simulink model "t06_manual_control_sol"  (R2024b)
settings: Solver=ode23t  StartTime=0.0  StopTime=inf  RelTol=1e-3  AbsTol=1e-3  EnableMultiTasking=on
model workspace (MAT data in the model file):
  A = 0.4
  Critical_Velocity = 0.01
  Damping_Factor = 1000
  Dynamic_Friction = 0.5
  Heigth_brick : Simulink.Parameter (value not decoded)
  Heigth_ramp : Simulink.Parameter (value not decoded)
  Length_brick : Simulink.Parameter (value not decoded)
  Length_ramp : Simulink.Parameter (value not decoded)
  Length_torso : Simulink.Parameter (value not decoded)
  Lower_limbs : Simulink.Parameter (value not decoded)
  Static_Friction = 0.7
  Stiffnesscoefficient = 10000
  Transition_Region_Width = 0.02
  Upper_limbs : Simulink.Parameter (value not decoded)
  Width_brick : Simulink.Parameter (value not decoded)
  Width_ramp : Simulink.Parameter (value not decoded)
  Width_torso : Simulink.Parameter (value not decoded)
  f = 1.5
  max_Joint_change = 100
  r_foot : Simulink.Parameter (value not decoded)
  sampleTime : Simulink.Parameter (value not decoded)
  t_leg : Simulink.Parameter (value not decoded)
  theta : Simulink.Parameter (value not decoded)
  transferFunVal : Simulink.Parameter (value not decoded)
symbols that are objects in the model workspace (value not decoded): Length_torso, Lower_limbs, t_leg, Upper_limbs, Width_torso
undefined symbols (not defined in the file): X, Y, Z
libraries: sm_lib x78, nesl_utility x13, functionAngles x6, functionBezier_backward x3, vrlib x1
(part 4 of 5)

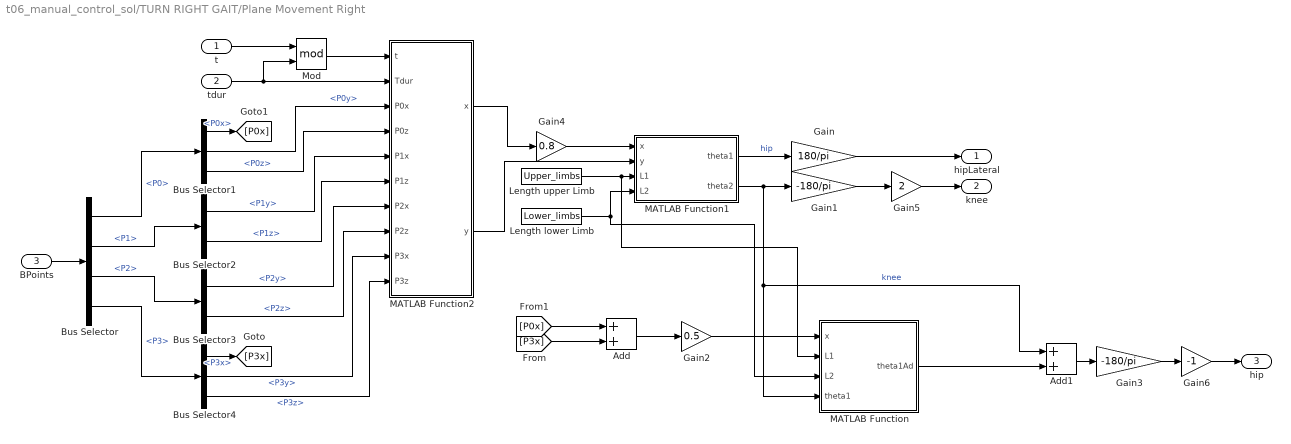
== system t06_manual_control_sol/TURN RIGHT GAIT/Plane Movement Right ==
  t : Inport
  tdur : Inport  Port=2
  BPoints : Inport  Port=3
  Add : Sum
  Add1 : Sum
  Bus Selector : BusSelector  OutputSignals=P0,P1,P2,P3
  Bus Selector1 : BusSelector  OutputSignals=P0x,P0y,P0z
  Bus Selector2 : BusSelector  OutputSignals=P1y,P1z
  Bus Selector3 : BusSelector  OutputSignals=P2y,P2z
  Bus Selector4 : BusSelector  OutputSignals=P3x,P3y,P3z
  Gain : Gain  Gain=180/pi
  Gain1 : Gain  Gain=-180/pi
  Gain2 : Gain  Gain=0.5
  Gain3 : Gain  Gain=-180/pi
  Gain4 : Gain  Gain=0.8
  Gain5 : Gain  Gain=2
  Gain6 : Gain  Gain=-1
  Length lower Limb : Constant  Value=Lower_limbs
  Length upper Limb : Constant  Value=Upper_limbs
  MATLAB Function : MATLAB Function  TreatAsAtomicUnit=on
  MATLAB Function1 : MATLAB Function  TreatAsAtomicUnit=on
  MATLAB Function2 : MATLAB Function  TreatAsAtomicUnit=on
  Mod : Math  Operator=mod
  hipLateral : Outport
  knee : Outport  Port=2
  hip : Outport  Port=3
  wires:
  Gain4/1 -> MATLAB Function1/1(x)
  Gain3/1 -> Gain6/1
  Add1/1 -> Gain3/1
  Bus Selector1/1 -> [P0x]  "<P0x>"
  Bus Selector4/1 -> [P3x]  "<P3x>"
  MATLAB Function/1(theta1Ad) -> Add1/2
  [P3x] -> Add/2
  [P0x] -> Add/1
  Add/1 -> Gain2/1
  Gain2/1 -> MATLAB Function/1(x)
  Gain/1 -> hipLateral/1
  Gain1/1 -> Gain5/1
  Length lower Limb/1 -> MATLAB Function1/4(L2), MATLAB Function/3(L2)
  Length upper Limb/1 -> MATLAB Function1/3(L1), MATLAB Function/2(L1)
  t/1 -> Mod/1
  MATLAB Function1/1(theta1) -> Gain/1  "hip"
  tdur/1 -> MATLAB Function2/2(Tdur), Mod/2
  MATLAB Function1/2(theta2) -> Gain1/1, MATLAB Function/4(theta1), Add1/1  "knee"
  MATLAB Function2/1(x) -> Gain4/1
  MATLAB Function2/2(y) -> MATLAB Function1/2(y)
  Bus Selector/3 -> Bus Selector3/1  "<P2>"
  Bus Selector3/2 -> MATLAB Function2/8(P2z)  "<P2z>"
  Bus Selector2/1 -> MATLAB Function2/5(P1x)  "<P1y>"
  Bus Selector3/1 -> MATLAB Function2/7(P2x)  "<P2y>"
  Bus Selector4/2 -> MATLAB Function2/9(P3x)  "<P3y>"
  Bus Selector1/3 -> MATLAB Function2/4(P0z)  "<P0z>"
  Bus Selector/4 -> Bus Selector4/1  "<P3>"
  Bus Selector4/3 -> MATLAB Function2/10(P3z)  "<P3z>"
  Bus Selector/2 -> Bus Selector2/1  "<P1>"
  BPoints/1 -> Bus Selector/1
  Bus Selector1/2 -> MATLAB Function2/3(P0x)  "<P0y>"
  Bus Selector/1 -> Bus Selector1/1  "<P0>"
  Bus Selector2/2 -> MATLAB Function2/6(P1z)  "<P1z>"
  Mod/1 -> MATLAB Function2/1(t)
  Gain5/1 -> knee/1
  Gain6/1 -> hip/1

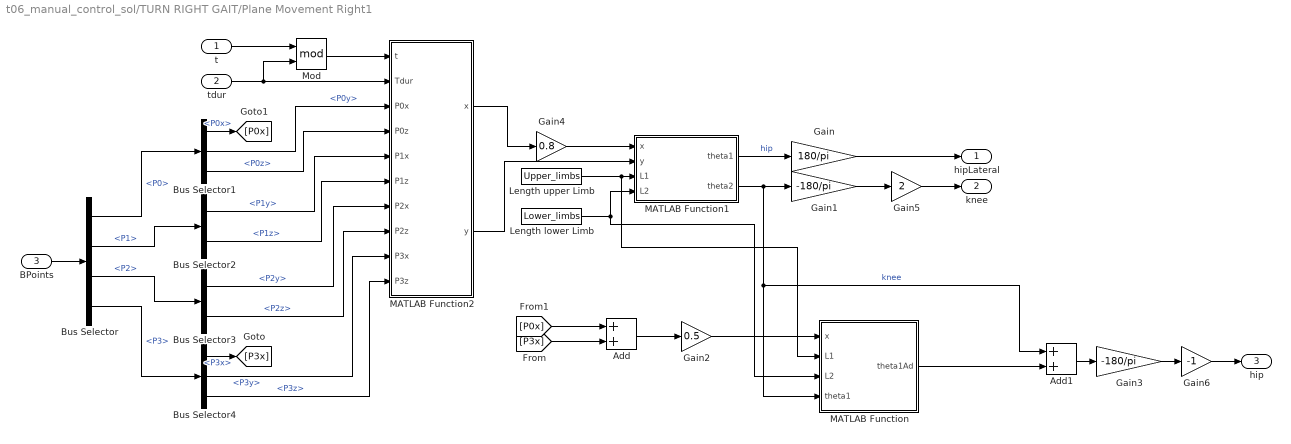
== system t06_manual_control_sol/TURN RIGHT GAIT/Plane Movement Right1 ==
  t : Inport
  tdur : Inport  Port=2
  BPoints : Inport  Port=3
  Add : Sum
  Add1 : Sum
  Bus Selector : BusSelector  OutputSignals=P0,P1,P2,P3
  Bus Selector1 : BusSelector  OutputSignals=P0x,P0y,P0z
  Bus Selector2 : BusSelector  OutputSignals=P1y,P1z
  Bus Selector3 : BusSelector  OutputSignals=P2y,P2z
  Bus Selector4 : BusSelector  OutputSignals=P3x,P3y,P3z
  Gain : Gain  Gain=180/pi
  Gain1 : Gain  Gain=-180/pi
  Gain2 : Gain  Gain=0.5
  Gain3 : Gain  Gain=-180/pi
  Gain4 : Gain  Gain=0.8
  Gain5 : Gain  Gain=2
  Gain6 : Gain  Gain=-1
  Length lower Limb : Constant  Value=Lower_limbs
  Length upper Limb : Constant  Value=Upper_limbs
  MATLAB Function : MATLAB Function  TreatAsAtomicUnit=on
  MATLAB Function1 : MATLAB Function  TreatAsAtomicUnit=on
  MATLAB Function2 : MATLAB Function  TreatAsAtomicUnit=on
  Mod : Math  Operator=mod
  hipLateral : Outport
  knee : Outport  Port=2
  hip : Outport  Port=3
  wires:
  Gain6/1 -> hip/1
  Gain5/1 -> knee/1
  Mod/1 -> MATLAB Function2/1(t)
  Bus Selector2/2 -> MATLAB Function2/6(P1z)  "<P1z>"
  Bus Selector/1 -> Bus Selector1/1  "<P0>"
  Bus Selector1/2 -> MATLAB Function2/3(P0x)  "<P0y>"
  BPoints/1 -> Bus Selector/1
  Bus Selector/2 -> Bus Selector2/1  "<P1>"
  Bus Selector4/3 -> MATLAB Function2/10(P3z)  "<P3z>"
  Bus Selector/4 -> Bus Selector4/1  "<P3>"
  Bus Selector1/3 -> MATLAB Function2/4(P0z)  "<P0z>"
  Bus Selector4/2 -> MATLAB Function2/9(P3x)  "<P3y>"
  Bus Selector3/1 -> MATLAB Function2/7(P2x)  "<P2y>"
  Bus Selector2/1 -> MATLAB Function2/5(P1x)  "<P1y>"
  Bus Selector3/2 -> MATLAB Function2/8(P2z)  "<P2z>"
  Bus Selector/3 -> Bus Selector3/1  "<P2>"
  MATLAB Function2/2(y) -> MATLAB Function1/2(y)
  MATLAB Function2/1(x) -> Gain4/1
  MATLAB Function1/2(theta2) -> Add1/1, MATLAB Function/4(theta1), Gain1/1  "knee"
  tdur/1 -> Mod/2, MATLAB Function2/2(Tdur)
  MATLAB Function1/1(theta1) -> Gain/1  "hip"
  t/1 -> Mod/1
  Length upper Limb/1 -> MATLAB Function/2(L1), MATLAB Function1/3(L1)
  Length lower Limb/1 -> MATLAB Function/3(L2), MATLAB Function1/4(L2)
  Gain1/1 -> Gain5/1
  Gain/1 -> hipLateral/1
  Gain2/1 -> MATLAB Function/1(x)
  Add/1 -> Gain2/1
  [P0x] -> Add/1
  [P3x] -> Add/2
  MATLAB Function/1(theta1Ad) -> Add1/2
  Bus Selector4/1 -> [P3x]  "<P3x>"
  Bus Selector1/1 -> [P0x]  "<P0x>"
  Add1/1 -> Gain3/1
  Gain3/1 -> Gain6/1
  Gain4/1 -> MATLAB Function1/1(x)

== system t06_manual_control_sol/TURN RIGHT GAIT/Subsystem ==
  t : Inport
  tdur : Inport  Port=2
  Add : Sum  Inputs=+-
  Add1 : Sum  Inputs=+-
  Add2 : Sum  Inputs=+-
  Gain : Gain  Gain=0.25
  Gain1 : Gain  Gain=0.5
  Gain2 : Gain  Gain=0.75
  t_0.25 : Outport
  t_0.5 : Outport  Port=2
  t_0.75 : Outport  Port=3
  wires:
  tdur/1 -> Gain/1, Gain2/1, Gain1/1
  Gain2/1 -> Add2/2
  Gain1/1 -> Add1/2
  t/1 -> Add/1, Add1/1, Add2/1
  Gain/1 -> Add/2
  Add/1 -> t_0.25/1
  Add1/1 -> t_0.5/1
  Add2/1 -> t_0.75/1

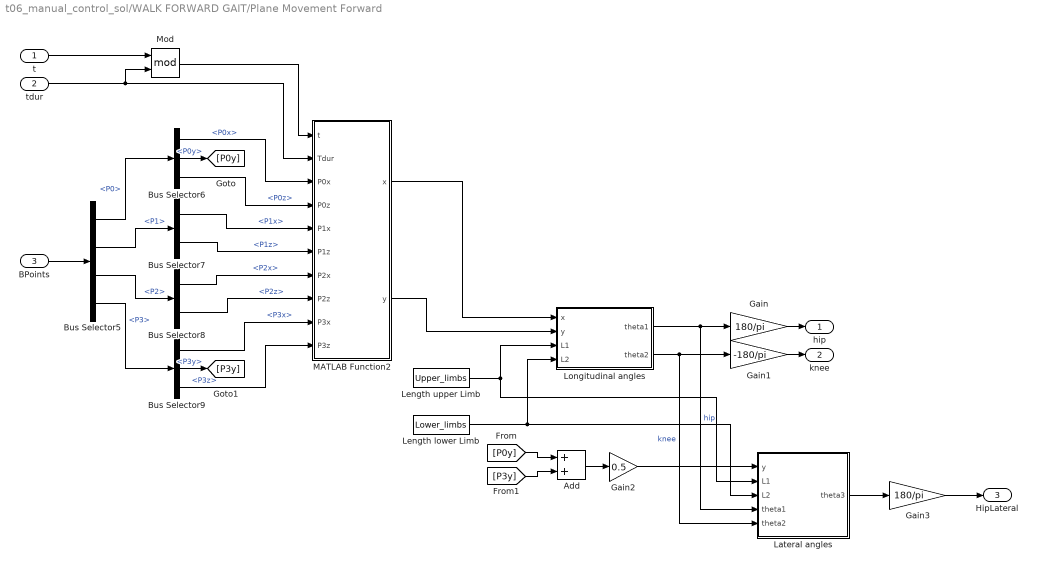
== system t06_manual_control_sol/WALK FORWARD GAIT/Plane Movement Forward ==
  t : Inport
  tdur : Inport  Port=2
  BPoints : Inport  Port=3
  Add : Sum
  Bus Selector5 : BusSelector  OutputSignals=P0,P1,P2,P3
  Bus Selector6 : BusSelector  OutputSignals=P0x,P0y,P0z
  Bus Selector7 : BusSelector  OutputSignals=P1x,P1z
  Bus Selector8 : BusSelector  OutputSignals=P2x,P2z
  Bus Selector9 : BusSelector  OutputSignals=P3x,P3y,P3z
  Gain : Gain  Gain=180/pi
  Gain1 : Gain  Gain=-180/pi
  Gain2 : Gain  Gain=0.5
  Gain3 : Gain  Gain=180/pi
  Lateral angles : MATLAB Function  TreatAsAtomicUnit=on
  Length lower Limb : Constant  Value=Lower_limbs
  Length upper Limb : Constant  Value=Upper_limbs
  Longitudinal angles : MATLAB Function  TreatAsAtomicUnit=on
  MATLAB Function2 : MATLAB Function  TreatAsAtomicUnit=on
  Mod : Math  Operator=mod
  hip : Outport
  knee : Outport  Port=2
  HipLateral : Outport  Port=3
  wires:
  Gain3/1 -> HipLateral/1
  Lateral angles/1(theta3) -> Gain3/1
  [P3y] -> Add/2
  [P0y] -> Add/1
  Bus Selector9/2 -> [P3y]  "<P3y>"
  Bus Selector6/2 -> [P0y]  "<P0y>"
  Gain2/1 -> Lateral angles/1(y)
  Add/1 -> Gain2/1
  Gain/1 -> hip/1
  Gain1/1 -> knee/1
  Length lower Limb/1 -> Lateral angles/3(L2), Longitudinal angles/4(L2)
  Length upper Limb/1 -> Lateral angles/2(L1), Longitudinal angles/3(L1)
  t/1 -> Mod/1
  Longitudinal angles/1(theta1) -> Gain/1, Lateral angles/4(theta1)  "hip"
  tdur/1 -> Mod/2, MATLAB Function2/2(Tdur)
  Longitudinal angles/2(theta2) -> Lateral angles/5(theta2), Gain1/1  "knee"
  MATLAB Function2/1(x) -> Longitudinal angles/1(x)
  MATLAB Function2/2(y) -> Longitudinal angles/2(y)
  Bus Selector5/3 -> Bus Selector8/1  "<P2>"
  Bus Selector8/2 -> MATLAB Function2/8(P2z)  "<P2z>"
  Bus Selector7/1 -> MATLAB Function2/5(P1x)  "<P1x>"
  Bus Selector8/1 -> MATLAB Function2/7(P2x)  "<P2x>"
  Bus Selector9/1 -> MATLAB Function2/9(P3x)  "<P3x>"
  Bus Selector6/3 -> MATLAB Function2/4(P0z)  "<P0z>"
  Bus Selector5/4 -> Bus Selector9/1  "<P3>"
  Bus Selector9/3 -> MATLAB Function2/10(P3z)  "<P3z>"
  Bus Selector5/2 -> Bus Selector7/1  "<P1>"
  BPoints/1 -> Bus Selector5/1
  Bus Selector6/1 -> MATLAB Function2/3(P0x)  "<P0x>"
  Bus Selector5/1 -> Bus Selector6/1  "<P0>"
  Bus Selector7/2 -> MATLAB Function2/6(P1z)  "<P1z>"
  Mod/1 -> MATLAB Function2/1(t)

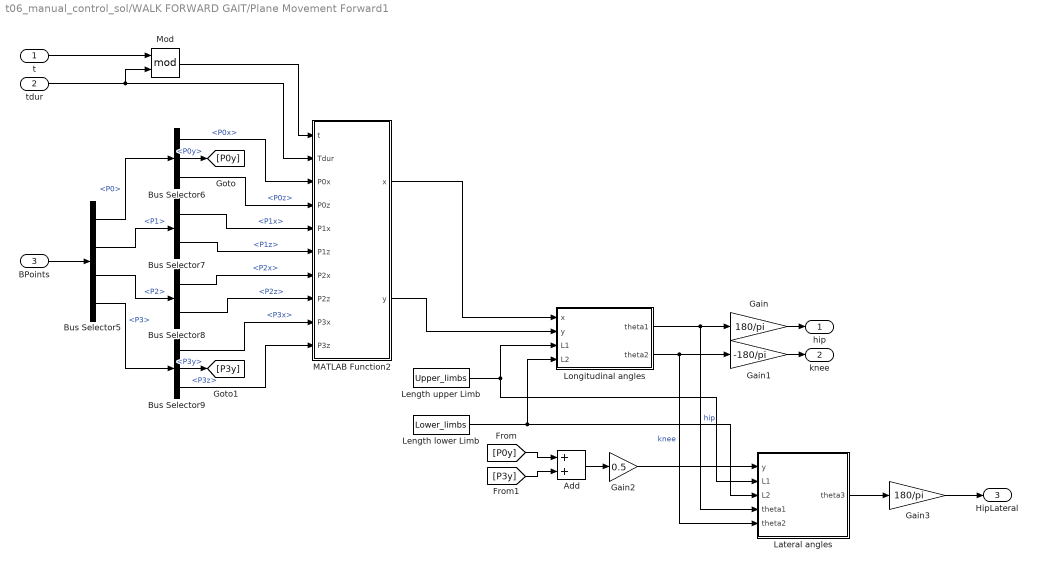
== system t06_manual_control_sol/WALK FORWARD GAIT/Plane Movement Forward1 ==
  t : Inport
  tdur : Inport  Port=2
  BPoints : Inport  Port=3
  Add : Sum
  Bus Selector5 : BusSelector  OutputSignals=P0,P1,P2,P3
  Bus Selector6 : BusSelector  OutputSignals=P0x,P0y,P0z
  Bus Selector7 : BusSelector  OutputSignals=P1x,P1z
  Bus Selector8 : BusSelector  OutputSignals=P2x,P2z
  Bus Selector9 : BusSelector  OutputSignals=P3x,P3y,P3z
  Gain : Gain  Gain=180/pi
  Gain1 : Gain  Gain=-180/pi
  Gain2 : Gain  Gain=0.5
  Gain3 : Gain  Gain=180/pi
  Lateral angles : MATLAB Function  TreatAsAtomicUnit=on
  Length lower Limb : Constant  Value=Lower_limbs
  Length upper Limb : Constant  Value=Upper_limbs
  Longitudinal angles : MATLAB Function  TreatAsAtomicUnit=on
  MATLAB Function2 : MATLAB Function  TreatAsAtomicUnit=on
  Mod : Math  Operator=mod
  hip : Outport
  knee : Outport  Port=2
  HipLateral : Outport  Port=3
  wires:
  Gain3/1 -> HipLateral/1
  Lateral angles/1(theta3) -> Gain3/1
  [P3y] -> Add/2
  [P0y] -> Add/1
  Bus Selector9/2 -> [P3y]  "<P3y>"
  Bus Selector6/2 -> [P0y]  "<P0y>"
  Gain2/1 -> Lateral angles/1(y)
  Add/1 -> Gain2/1
  Gain/1 -> hip/1
  Gain1/1 -> knee/1
  Length lower Limb/1 -> Lateral angles/3(L2), Longitudinal angles/4(L2)
  Length upper Limb/1 -> Lateral angles/2(L1), Longitudinal angles/3(L1)
  t/1 -> Mod/1
  Longitudinal angles/1(theta1) -> Gain/1, Lateral angles/4(theta1)  "hip"
  tdur/1 -> Mod/2, MATLAB Function2/2(Tdur)
  Longitudinal angles/2(theta2) -> Lateral angles/5(theta2), Gain1/1  "knee"
  MATLAB Function2/1(x) -> Longitudinal angles/1(x)
  MATLAB Function2/2(y) -> Longitudinal angles/2(y)
  Bus Selector5/3 -> Bus Selector8/1  "<P2>"
  Bus Selector8/2 -> MATLAB Function2/8(P2z)  "<P2z>"
  Bus Selector7/1 -> MATLAB Function2/5(P1x)  "<P1x>"
  Bus Selector8/1 -> MATLAB Function2/7(P2x)  "<P2x>"
  Bus Selector9/1 -> MATLAB Function2/9(P3x)  "<P3x>"
  Bus Selector6/3 -> MATLAB Function2/4(P0z)  "<P0z>"
  Bus Selector5/4 -> Bus Selector9/1  "<P3>"
  Bus Selector9/3 -> MATLAB Function2/10(P3z)  "<P3z>"
  Bus Selector5/2 -> Bus Selector7/1  "<P1>"
  BPoints/1 -> Bus Selector5/1
  Bus Selector6/1 -> MATLAB Function2/3(P0x)  "<P0x>"
  Bus Selector5/1 -> Bus Selector6/1  "<P0>"
  Bus Selector7/2 -> MATLAB Function2/6(P1z)  "<P1z>"
  Mod/1 -> MATLAB Function2/1(t)

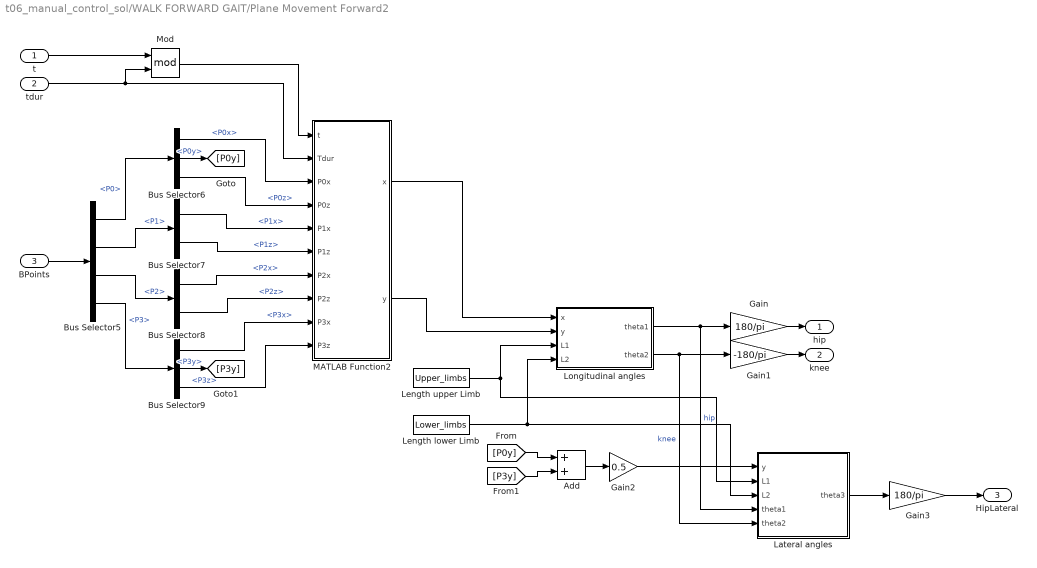
== system t06_manual_control_sol/WALK FORWARD GAIT/Plane Movement Forward2 ==
  t : Inport
  tdur : Inport  Port=2
  BPoints : Inport  Port=3
  Add : Sum
  Bus Selector5 : BusSelector  OutputSignals=P0,P1,P2,P3
  Bus Selector6 : BusSelector  OutputSignals=P0x,P0y,P0z
  Bus Selector7 : BusSelector  OutputSignals=P1x,P1z
  Bus Selector8 : BusSelector  OutputSignals=P2x,P2z
  Bus Selector9 : BusSelector  OutputSignals=P3x,P3y,P3z
  Gain : Gain  Gain=180/pi
  Gain1 : Gain  Gain=-180/pi
  Gain2 : Gain  Gain=0.5
  Gain3 : Gain  Gain=180/pi
  Lateral angles : MATLAB Function  TreatAsAtomicUnit=on
  Length lower Limb : Constant  Value=Lower_limbs
  Length upper Limb : Constant  Value=Upper_limbs
  Longitudinal angles : MATLAB Function  TreatAsAtomicUnit=on
  MATLAB Function2 : MATLAB Function  TreatAsAtomicUnit=on
  Mod : Math  Operator=mod
  hip : Outport
  knee : Outport  Port=2
  HipLateral : Outport  Port=3
  wires:
  Gain3/1 -> HipLateral/1
  Lateral angles/1(theta3) -> Gain3/1
  [P3y] -> Add/2
  [P0y] -> Add/1
  Bus Selector9/2 -> [P3y]  "<P3y>"
  Bus Selector6/2 -> [P0y]  "<P0y>"
  Gain2/1 -> Lateral angles/1(y)
  Add/1 -> Gain2/1
  Gain/1 -> hip/1
  Gain1/1 -> knee/1
  Length lower Limb/1 -> Lateral angles/3(L2), Longitudinal angles/4(L2)
  Length upper Limb/1 -> Lateral angles/2(L1), Longitudinal angles/3(L1)
  t/1 -> Mod/1
  Longitudinal angles/1(theta1) -> Gain/1, Lateral angles/4(theta1)  "hip"
  tdur/1 -> Mod/2, MATLAB Function2/2(Tdur)
  Longitudinal angles/2(theta2) -> Lateral angles/5(theta2), Gain1/1  "knee"
  MATLAB Function2/1(x) -> Longitudinal angles/1(x)
  MATLAB Function2/2(y) -> Longitudinal angles/2(y)
  Bus Selector5/3 -> Bus Selector8/1  "<P2>"
  Bus Selector8/2 -> MATLAB Function2/8(P2z)  "<P2z>"
  Bus Selector7/1 -> MATLAB Function2/5(P1x)  "<P1x>"
  Bus Selector8/1 -> MATLAB Function2/7(P2x)  "<P2x>"
  Bus Selector9/1 -> MATLAB Function2/9(P3x)  "<P3x>"
  Bus Selector6/3 -> MATLAB Function2/4(P0z)  "<P0z>"
  Bus Selector5/4 -> Bus Selector9/1  "<P3>"
  Bus Selector9/3 -> MATLAB Function2/10(P3z)  "<P3z>"
  Bus Selector5/2 -> Bus Selector7/1  "<P1>"
  BPoints/1 -> Bus Selector5/1
  Bus Selector6/1 -> MATLAB Function2/3(P0x)  "<P0x>"
  Bus Selector5/1 -> Bus Selector6/1  "<P0>"
  Bus Selector7/2 -> MATLAB Function2/6(P1z)  "<P1z>"
  Mod/1 -> MATLAB Function2/1(t)

== system t06_manual_control_sol/WALK FORWARD GAIT/Plane Movement Forward3 ==
  t : Inport
  tdur : Inport  Port=2
  BPoints : Inport  Port=3
  Add : Sum
  Bus Selector5 : BusSelector  OutputSignals=P0,P1,P2,P3
  Bus Selector6 : BusSelector  OutputSignals=P0x,P0y,P0z
  Bus Selector7 : BusSelector  OutputSignals=P1x,P1z
  Bus Selector8 : BusSelector  OutputSignals=P2x,P2z
  Bus Selector9 : BusSelector  OutputSignals=P3x,P3y,P3z
  Gain : Gain  Gain=180/pi
  Gain1 : Gain  Gain=-180/pi
  Gain2 : Gain  Gain=0.5
  Gain3 : Gain  Gain=180/pi
  Lateral angles : MATLAB Function  TreatAsAtomicUnit=on
  Length lower Limb : Constant  Value=Lower_limbs
  Length upper Limb : Constant  Value=Upper_limbs
  Longitudinal angles : MATLAB Function  TreatAsAtomicUnit=on
  MATLAB Function2 : MATLAB Function  TreatAsAtomicUnit=on
  Mod : Math  Operator=mod
  hip : Outport
  knee : Outport  Port=2
  HipLateral : Outport  Port=3
  wires:
  Gain3/1 -> HipLateral/1
  Lateral angles/1(theta3) -> Gain3/1
  [P3y] -> Add/2
  [P0y] -> Add/1
  Bus Selector9/2 -> [P3y]  "<P3y>"
  Bus Selector6/2 -> [P0y]  "<P0y>"
  Gain2/1 -> Lateral angles/1(y)
  Add/1 -> Gain2/1
  Gain/1 -> hip/1
  Gain1/1 -> knee/1
  Length lower Limb/1 -> Lateral angles/3(L2), Longitudinal angles/4(L2)
  Length upper Limb/1 -> Lateral angles/2(L1), Longitudinal angles/3(L1)
  t/1 -> Mod/1
  Longitudinal angles/1(theta1) -> Gain/1, Lateral angles/4(theta1)  "hip"
  tdur/1 -> Mod/2, MATLAB Function2/2(Tdur)
  Longitudinal angles/2(theta2) -> Lateral angles/5(theta2), Gain1/1  "knee"
  MATLAB Function2/1(x) -> Longitudinal angles/1(x)
  MATLAB Function2/2(y) -> Longitudinal angles/2(y)
  Bus Selector5/3 -> Bus Selector8/1  "<P2>"
  Bus Selector8/2 -> MATLAB Function2/8(P2z)  "<P2z>"
  Bus Selector7/1 -> MATLAB Function2/5(P1x)  "<P1x>"
  Bus Selector8/1 -> MATLAB Function2/7(P2x)  "<P2x>"
  Bus Selector9/1 -> MATLAB Function2/9(P3x)  "<P3x>"
  Bus Selector6/3 -> MATLAB Function2/4(P0z)  "<P0z>"
  Bus Selector5/4 -> Bus Selector9/1  "<P3>"
  Bus Selector9/3 -> MATLAB Function2/10(P3z)  "<P3z>"
  Bus Selector5/2 -> Bus Selector7/1  "<P1>"
  BPoints/1 -> Bus Selector5/1
  Bus Selector6/1 -> MATLAB Function2/3(P0x)  "<P0x>"
  Bus Selector5/1 -> Bus Selector6/1  "<P0>"
  Bus Selector7/2 -> MATLAB Function2/6(P1z)  "<P1z>"
  Mod/1 -> MATLAB Function2/1(t)

== system t06_manual_control_sol/WALK FORWARD GAIT/Subsystem ==
  t : Inport
  tdur : Inport  Port=2
  Add : Sum  Inputs=+-
  Add1 : Sum  Inputs=+-
  Add2 : Sum  Inputs=+-
  Gain : Gain  Gain=0.25
  Gain1 : Gain  Gain=0.5
  Gain2 : Gain  Gain=0.75
  t_0.25 : Outport
  t_0.5 : Outport  Port=2
  t_0.75 : Outport  Port=3
  wires:
  tdur/1 -> Gain/1, Gain2/1, Gain1/1
  Gain2/1 -> Add2/2
  Gain1/1 -> Add1/2
  t/1 -> Add/1, Add1/1, Add2/1
  Gain/1 -> Add/2
  Add/1 -> t_0.25/1
  Add1/1 -> t_0.5/1
  Add2/1 -> t_0.75/1

== system t06_manual_control_sol/Walk Back Gait - Bezier Curves/Plane Movement BL ==
  t : Inport
  tdur : Inport  Port=2
  BPoints : Inport  Port=3
  Add : Sum
  Bus Selector : BusSelector  OutputSignals=P0,P1,P2,P3
  Bus Selector1 : BusSelector  OutputSignals=P0x,P0y,P0z
  Bus Selector2 : BusSelector  OutputSignals=P1x,P1z
  Bus Selector3 : BusSelector  OutputSignals=P2x,P2z
  Bus Selector4 : BusSelector  OutputSignals=P3x,P3y,P3z
  Gain : Gain  Gain=180/pi
  Gain1 : Gain  Gain=-180/pi
  Gain2 : Gain  Gain=0.5
  Gain3 : Gain  Gain=180/pi
  Length lower Limb : Constant  Value=Lower_limbs
  Length upper Limb : Constant  Value=Upper_limbs
  MATLAB : functionAngles/MATLAB  SystemSampleTime=-1  VariantActivationTime=update diagram  AllowFlexibleInterface=on  Latency=0  AutoFrameSizeCalculation=off
  MATLAB Function : functionAngles/MATLAB Function  SystemSampleTime=-1  VariantActivationTime=update diagram  AllowFlexibleInterface=on  Latency=0  AutoFrameSizeCalculation=off
  MATLAB Function2 : functionBezier_backward/MATLAB Function2  SystemSampleTime=-1  VariantActivationTime=update diagram  AllowFlexibleInterface=on  Latency=0  AutoFrameSizeCalculation=off
  Mod : Math  Operator=mod
  hip : Outport
  knee : Outport  Port=2
  hipLateral : Outport  Port=3
  wires:
  MATLAB Function/1 -> Gain3/1
  Gain3/1 -> hipLateral/1
  Bus Selector4/2 -> [P3y]  "<P3y>"
  Bus Selector1/2 -> [P0y]  "<P0y>"
  Gain2/1 -> MATLAB Function/1
  [P3y] -> Add/2
  Add/1 -> Gain2/1
  [P0y] -> Add/1
  MATLAB Function2/2 -> MATLAB/2
  MATLAB Function2/1 -> MATLAB/1
  MATLAB/2 -> Gain1/1, MATLAB Function/5  "knee"
  tdur/1 -> Mod/2, MATLAB Function2/2
  MATLAB/1 -> Gain/1, MATLAB Function/4  "hip"
  Length upper Limb/1 -> MATLAB Function/2, MATLAB/3
  Length lower Limb/1 -> MATLAB/4, MATLAB Function/3
  Gain1/1 -> knee/1
  Gain/1 -> hip/1
  Bus Selector/3 -> Bus Selector3/1  "<P2>"
  Bus Selector3/2 -> MATLAB Function2/8  "<P2z>"
  Bus Selector2/1 -> MATLAB Function2/5  "<P1x>"
  Bus Selector3/1 -> MATLAB Function2/7  "<P2x>"
  Bus Selector4/1 -> MATLAB Function2/9  "<P3x>"
  Bus Selector1/3 -> MATLAB Function2/4  "<P0z>"
  Bus Selector/4 -> Bus Selector4/1  "<P3>"
  Bus Selector4/3 -> MATLAB Function2/10  "<P3z>"
  Bus Selector/2 -> Bus Selector2/1  "<P1>"
  BPoints/1 -> Bus Selector/1
  Bus Selector1/1 -> MATLAB Function2/3  "<P0x>"
  Bus Selector/1 -> Bus Selector1/1  "<P0>"
  Bus Selector2/2 -> MATLAB Function2/6  "<P1z>"
  t/1 -> Mod/1
  Mod/1 -> MATLAB Function2/1

== system t06_manual_control_sol/Walk Back Gait - Bezier Curves/Plane Movement BR ==
  t : Inport
  tdur : Inport  Port=2
  BPoints : Inport  Port=3
  Add : Sum
  Bus Selector : BusSelector  OutputSignals=P0,P1,P2,P3
  Bus Selector1 : BusSelector  OutputSignals=P0x,P0y,P0z
  Bus Selector2 : BusSelector  OutputSignals=P1x,P1z
  Bus Selector3 : BusSelector  OutputSignals=P2x,P2z
  Bus Selector4 : BusSelector  OutputSignals=P3x,P3y,P3z
  Gain : Gain  Gain=180/pi
  Gain1 : Gain  Gain=-180/pi
  Gain2 : Gain  Gain=0.5
  Gain3 : Gain  Gain=180/pi
  Length lower Limb : Constant  Value=Lower_limbs
  Length upper Limb : Constant  Value=Upper_limbs
  MATLAB : functionAngles/MATLAB  SystemSampleTime=-1  VariantActivationTime=update diagram  AllowFlexibleInterface=on  Latency=0  AutoFrameSizeCalculation=off
  MATLAB Function : functionAngles/MATLAB Function  SystemSampleTime=-1  VariantActivationTime=update diagram  AllowFlexibleInterface=on  Latency=0  AutoFrameSizeCalculation=off
  MATLAB Function2 : functionBezier_backward/MATLAB Function2  SystemSampleTime=-1  VariantActivationTime=update diagram  AllowFlexibleInterface=on  Latency=0  AutoFrameSizeCalculation=off
  Mod : Math  Operator=mod
  hip : Outport
  knee : Outport  Port=2
  hipLateral : Outport  Port=3
  wires:
  MATLAB Function/1 -> Gain3/1
  Gain3/1 -> hipLateral/1
  Bus Selector4/2 -> [P3y]  "<P3y>"
  Bus Selector1/2 -> [P0y]  "<P0y>"
  Gain2/1 -> MATLAB Function/1
  [P3y] -> Add/2
  Add/1 -> Gain2/1
  [P0y] -> Add/1
  MATLAB Function2/2 -> MATLAB/2
  MATLAB Function2/1 -> MATLAB/1
  MATLAB/2 -> Gain1/1, MATLAB Function/5  "knee"
  tdur/1 -> MATLAB Function2/2, Mod/2
  MATLAB/1 -> Gain/1, MATLAB Function/4  "hip"
  Length upper Limb/1 -> MATLAB Function/2, MATLAB/3
  Length lower Limb/1 -> MATLAB/4, MATLAB Function/3
  Gain1/1 -> knee/1
  Gain/1 -> hip/1
  Bus Selector/3 -> Bus Selector3/1  "<P2>"
  Bus Selector3/2 -> MATLAB Function2/8  "<P2z>"
  Bus Selector2/1 -> MATLAB Function2/5  "<P1x>"
  Bus Selector3/1 -> MATLAB Function2/7  "<P2x>"
  Bus Selector4/1 -> MATLAB Function2/9  "<P3x>"
  Bus Selector1/3 -> MATLAB Function2/4  "<P0z>"
  Bus Selector/4 -> Bus Selector4/1  "<P3>"
  Bus Selector4/3 -> MATLAB Function2/10  "<P3z>"
  Bus Selector/2 -> Bus Selector2/1  "<P1>"
  BPoints/1 -> Bus Selector/1
  Bus Selector1/1 -> MATLAB Function2/3  "<P0x>"
  Bus Selector/1 -> Bus Selector1/1  "<P0>"
  Bus Selector2/2 -> MATLAB Function2/6  "<P1z>"
  t/1 -> Mod/1
  Mod/1 -> MATLAB Function2/1

== system t06_manual_control_sol/Walk Back Gait - Bezier Curves/Plane Movement FL ==
  t : Inport
  tdur : Inport  Port=2
  BPoints : Inport  Port=3
  Add : Sum
  Bus Selector : BusSelector  OutputSignals=P0,P1,P2,P3
  Bus Selector1 : BusSelector  OutputSignals=P0x,P0y,P0z
  Bus Selector2 : BusSelector  OutputSignals=P1x,P1z
  Bus Selector3 : BusSelector  OutputSignals=P2x,P2z
  Bus Selector4 : BusSelector  OutputSignals=P3x,P3y,P3z
  Gain : Gain  Gain=180/pi
  Gain1 : Gain  Gain=-180/pi
  Gain2 : Gain  Gain=0.5
  Gain3 : Gain  Gain=180/pi
  Length lower Limb : Constant  Value=Lower_limbs
  Length upper Limb : Constant  Value=Upper_limbs
  MATLAB : MATLAB Function  TreatAsAtomicUnit=on
  MATLAB Function : MATLAB Function  TreatAsAtomicUnit=on
  MATLAB Function2 : MATLAB Function  TreatAsAtomicUnit=on
  Mod : Math  Operator=mod
  hip : Outport
  knee : Outport  Port=2
  hipLateral : Outport  Port=3
  wires:
  MATLAB Function/1(theta3) -> Gain3/1
  Gain3/1 -> hipLateral/1
  Bus Selector4/2 -> [P3y]  "<P3y>"
  Bus Selector1/2 -> [P0y]  "<P0y>"
  Gain2/1 -> MATLAB Function/1(y)
  [P3y] -> Add/2
  Add/1 -> Gain2/1
  [P0y] -> Add/1
  MATLAB Function2/2(y) -> MATLAB/2(y)
  MATLAB Function2/1(x) -> MATLAB/1(x)
  MATLAB/2(theta2) -> Gain1/1, MATLAB Function/5(theta2)  "knee"
  tdur/1 -> Mod/2, MATLAB Function2/2(Tdur)
  MATLAB/1(theta1) -> Gain/1, MATLAB Function/4(theta1)  "hip"
  Length upper Limb/1 -> MATLAB Function/2(L1), MATLAB/3(L1)
  Length lower Limb/1 -> MATLAB/4(L2), MATLAB Function/3(L2)
  Gain1/1 -> knee/1
  Gain/1 -> hip/1
  Bus Selector/3 -> Bus Selector3/1  "<P2>"
  Bus Selector3/2 -> MATLAB Function2/8(P2z)  "<P2z>"
  Bus Selector2/1 -> MATLAB Function2/5(P1x)  "<P1x>"
  Bus Selector3/1 -> MATLAB Function2/7(P2x)  "<P2x>"
  Bus Selector4/1 -> MATLAB Function2/9(P3x)  "<P3x>"
  Bus Selector1/3 -> MATLAB Function2/4(P0z)  "<P0z>"
  Bus Selector/4 -> Bus Selector4/1  "<P3>"
  Bus Selector4/3 -> MATLAB Function2/10(P3z)  "<P3z>"
  Bus Selector/2 -> Bus Selector2/1  "<P1>"
  BPoints/1 -> Bus Selector/1
  Bus Selector1/1 -> MATLAB Function2/3(P0x)  "<P0x>"
  Bus Selector/1 -> Bus Selector1/1  "<P0>"
  Bus Selector2/2 -> MATLAB Function2/6(P1z)  "<P1z>"
  Mod/1 -> MATLAB Function2/1(t)
  t/1 -> Mod/1

== system t06_manual_control_sol/Walk Back Gait - Bezier Curves/Plane Movement FR ==
  t : Inport
  tdur : Inport  Port=2
  BPoints : Inport  Port=3
  Add : Sum
  Bus Selector : BusSelector  OutputSignals=P0,P1,P2,P3
  Bus Selector1 : BusSelector  OutputSignals=P0x,P0y,P0z
  Bus Selector2 : BusSelector  OutputSignals=P1x,P1z
  Bus Selector3 : BusSelector  OutputSignals=P2x,P2z
  Bus Selector4 : BusSelector  OutputSignals=P3x,P3y,P3z
  Gain : Gain  Gain=180/pi
  Gain1 : Gain  Gain=-180/pi
  Gain2 : Gain  Gain=0.5
  Gain3 : Gain  Gain=180/pi
  Length lower Limb : Constant  Value=Lower_limbs
  Length upper Limb : Constant  Value=Upper_limbs
  MATLAB : functionAngles/MATLAB  SystemSampleTime=-1  VariantActivationTime=update diagram  AllowFlexibleInterface=on  Latency=0  AutoFrameSizeCalculation=off
  MATLAB Function : functionAngles/MATLAB Function  SystemSampleTime=-1  VariantActivationTime=update diagram  AllowFlexibleInterface=on  Latency=0  AutoFrameSizeCalculation=off
  MATLAB Function2 : functionBezier_backward/MATLAB Function2  SystemSampleTime=-1  VariantActivationTime=update diagram  AllowFlexibleInterface=on  Latency=0  AutoFrameSizeCalculation=off
  Mod : Math  Operator=mod
  hip : Outport
  knee : Outport  Port=2
  hipLateral : Outport  Port=3
  wires:
  MATLAB Function/1 -> Gain3/1
  Gain3/1 -> hipLateral/1
  Bus Selector4/2 -> [P3y]  "<P3y>"
  Bus Selector1/2 -> [P0y]  "<P0y>"
  Gain2/1 -> MATLAB Function/1
  [P3y] -> Add/2
  Add/1 -> Gain2/1
  [P0y] -> Add/1
  MATLAB Function2/2 -> MATLAB/2
  MATLAB Function2/1 -> MATLAB/1
  MATLAB/2 -> Gain1/1, MATLAB Function/5  "knee"
  tdur/1 -> Mod/2, MATLAB Function2/2
  MATLAB/1 -> Gain/1, MATLAB Function/4  "hip"
  Length upper Limb/1 -> MATLAB Function/2, MATLAB/3
  Length lower Limb/1 -> MATLAB/4, MATLAB Function/3
  Gain1/1 -> knee/1
  Gain/1 -> hip/1
  Bus Selector/3 -> Bus Selector3/1  "<P2>"
  Bus Selector3/2 -> MATLAB Function2/8  "<P2z>"
  Bus Selector2/1 -> MATLAB Function2/5  "<P1x>"
  Bus Selector3/1 -> MATLAB Function2/7  "<P2x>"
  Bus Selector4/1 -> MATLAB Function2/9  "<P3x>"
  Bus Selector1/3 -> MATLAB Function2/4  "<P0z>"
  Bus Selector/4 -> Bus Selector4/1  "<P3>"
  Bus Selector4/3 -> MATLAB Function2/10  "<P3z>"
  Bus Selector/2 -> Bus Selector2/1  "<P1>"
  BPoints/1 -> Bus Selector/1
  Bus Selector1/1 -> MATLAB Function2/3  "<P0x>"
  Bus Selector/1 -> Bus Selector1/1  "<P0>"
  Bus Selector2/2 -> MATLAB Function2/6  "<P1z>"
  t/1 -> Mod/1
  Mod/1 -> MATLAB Function2/1

== system t06_manual_control_sol/Walk Back Gait - Bezier Curves/Subsystem1 ==
  t : Inport
  tdur : Inport  Port=2
  Add : Sum  Inputs=+-
  Add1 : Sum  Inputs=+-
  Add2 : Sum  Inputs=+-
  Gain : Gain  Gain=0.25
  Gain1 : Gain  Gain=0.5
  Gain2 : Gain  Gain=0.75
  t_0.25 : Outport
  t_0.5 : Outport  Port=2
  t_0.75 : Outport  Port=3
  wires:
  tdur/1 -> Gain/1, Gain2/1, Gain1/1
  Gain2/1 -> Add2/2
  Gain1/1 -> Add1/2
  t/1 -> Add/1, Add1/1, Add2/1
  Gain/1 -> Add/2
  Add/1 -> t_0.25/1
  Add1/1 -> t_0.5/1
  Add2/1 -> t_0.75/1

== matlab function t06_manual_control_sol/TURN RIGHT GAIT/Plane Movement Left1/MATLAB Function1 ==
  data: x input; theta1 output; y input; L1 input; L2 input; theta2 output
function [theta1, theta2] = angSide(x,y,L1,L2)
theta1 = atan(-x/y);
if theta1 ~= 0
    d = x / (2*sin(theta1));
    theta2 = acos(d/L1);
else
    d = -y/2;
    theta2 = acos(d/L1);
end
end

== matlab function t06_manual_control_sol/WALK FORWARD GAIT/Plane Movement Forward1/Lateral angles ==
  data: y input; theta3 output; L1 input; L2 input; theta1 input; theta2 input
function theta3 = latAng(y, L1, L2, theta1, theta2)

l = cos(theta1)*(L1 + L2*cos(theta2));

theta3 = asin(y/l);

== matlab function t06_manual_control_sol/Stand Still/Plane Movement BL/Longitudinal angles ==
  data: x input; theta1 output; y input; L1 input; L2 input; theta2 output
function [theta1, theta2] = ang(x,y,L1,L2)
x;
y;
(x.^2+y.^2-L1.^2-L2.^2) / (2*L1*L2);
theta2 = acos((x.^2+y.^2-L1.^2-L2.^2) / (2*L1*L2));
beta = asin((L2*sin(theta2))./((x.^2+y.^2).^0.5));
theta1 = asin(x./((x.^2+y.^2).^0.5)) + beta;
end

== matlab function t06_manual_control_sol/Stand Still/Plane Movement BL/Lateral joint angle ==
  data: y input; theta3 output; L1 input; L2 input; theta1 input; theta2 input
function theta3 = latAng(y, L1, L2, theta1, theta2)

l = cos(theta1)*(L1 + L2*cos(theta2));

theta3 = asin(y/l);

== matlab function t06_manual_control_sol/Stand Still/Plane Movement BR/Longitudinal angles ==
  data: x input; theta1 output; y input; L1 input; L2 input; theta2 output
function [theta1, theta2] = ang(x,y,L1,L2)
x;
y;
(x.^2+y.^2-L1.^2-L2.^2) / (2*L1*L2);
theta2 = acos((x.^2+y.^2-L1.^2-L2.^2) / (2*L1*L2));
beta = asin((L2*sin(theta2))./((x.^2+y.^2).^0.5));
theta1 = asin(x./((x.^2+y.^2).^0.5)) + beta;
end

== matlab function t06_manual_control_sol/Stand Still/Plane Movement BR/Lateral joint angle ==
  data: y input; theta3 output; L1 input; L2 input; theta1 input; theta2 input
function theta3 = latAng(y, L1, L2, theta1, theta2)

l = cos(theta1)*(L1 + L2*cos(theta2));

theta3 = asin(y/l);

== matlab function t06_manual_control_sol/TURN RIGHT GAIT/Plane Movement Right1/MATLAB Function ==
  data: x input; theta1Ad output; L1 input; L2 input; theta1 input
function theta1Ad = angAd(x, L1, L2, theta1)

l = cos(theta1)*(L1 + L2);

theta1Ad = asin(-x/l);

== matlab function t06_manual_control_sol/Stand Still/Plane Movement FL/Lateral joint angle ==
  data: y input; theta3 output; L1 input; L2 input; theta1 input; theta2 input
function theta3 = latAng(y, L1, L2, theta1, theta2)

l = cos(theta1)*(L1 + L2*cos(theta2));

theta3 = asin(y/l);

== matlab function t06_manual_control_sol/Stand Still/Plane Movement FR/Lateral joint angle ==
  data: y input; theta3 output; L1 input; L2 input; theta1 input; theta2 input
function theta3 = latAng(y, L1, L2, theta1, theta2)

l = cos(theta1)*(L1 + L2*cos(theta2));

theta3 = asin(y/l);

== matlab function t06_manual_control_sol/Stand Still/Plane Movement FR/Longitudinal angles ==
  data: x input; theta1 output; y input; L1 input; L2 input; theta2 output
function [theta1, theta2] = ang(x,y,L1,L2)
x;
y;
(x.^2+y.^2-L1.^2-L2.^2) / (2*L1*L2);
theta2 = acos((x.^2+y.^2-L1.^2-L2.^2) / (2*L1*L2));
beta = asin((L2*sin(theta2))./((x.^2+y.^2).^0.5));
theta1 = asin(x./((x.^2+y.^2).^0.5)) + beta;
end

== matlab function t06_manual_control_sol/MATLAB Function1 ==
  data: u input; out output
function out = jsReadAxes(u)

out = 0;

if max(abs(u(1:2))) > 0.2

    if abs(u(1)) > abs(u(2)) % turning
        if u(1) < 0
            out = 2; % left
        else
            out = 3; % right
        end
    elseif abs(u(1)) < abs(u(2)) % walking
        if u(2) < 0
            out = 1; % front
        else
            out = 4; % backwards
        end
    end

end

end

== matlab function t06_manual_control_sol/MATLAB Function ==
  data: u input; out output
function out = jsReadButtons(u)

out = 0;
posVec = 0;

for i = 1:length(u)
    if u(i) == 1
        posVec = i;
    end
    
if posVec == 1 % walk backwards
    out = 4;
elseif posVec == 4 % walk forwards
    out = 1;
elseif posVec == 3 % turn left
    out = 2;
elseif posVec == 2 % turn right
    out = 3;

end
end

== matlab function t06_manual_control_sol/TURN RIGHT GAIT/Plane Movement Left1/MATLAB Function3 ==
  data: x output; t input; Tdur input; y output; P0x input; P0z input; P1x input; P1z input; P2x input; P2z input; P3x input; P3z input
function [x, y] = bez_plane_TrajV2(t,Tdur,P0x,P0z,P1x,P1z,P2x,P2z,P3x,P3z)
t_swing = Tdur/4;
t_support = Tdur*3/4;

P0 = [P0x, P0z];
P1 = [P1x, P1z];
P2 = [P2x, P2z];
P3 = [P3x, P3z];
P_ini = (P0 + P3)/2;

if Tdur == 0
    x = -P_ini(1);
    y = P_ini(2);

elseif t<=t_support/2
    x = -1*(P_ini(1)+(P3(1)-P0(1))/t_support*(t));
    y = P_ini(2);

elseif t<=t_support/2+t_swing
    t_ef = (t-t_support/2);
    Sw = P3*((1-(t_ef/t_swing))^3) + 3*P2*(t_ef/t_swing)*((1-(t_ef/t_swing))^2)...
        + 3*P1*((t_ef/t_swing)^2)*(1-(t_ef/t_swing)) + P0*((t_ef/t_swing)^3);
    
    x = -1*Sw(1);
    y = Sw(2);
else
    t_ef = (t-t_support/2-t_swing);
    x = -1*(P0(1)+(P3(1)-P0(1))/t_support*t_ef);
    y = P0(2);
end
end

== matlab function t06_manual_control_sol/TURN LEFT GAIT/Plane Movement Right1/MATLAB Function ==
  data: x input; theta1Ad output; L1 input; L2 input; theta1 input
function theta1Ad = angAd(x, L1, L2, theta1)

l = cos(theta1)*(L1 + L2);

theta1Ad = asin(-x/l);

== matlab function t06_manual_control_sol/TURN LEFT GAIT/Plane Movement Right1/MATLAB Function1 ==
  data: x input; theta1 output; y input; L1 input; L2 input; theta2 output
function [theta1, theta2] = angSide(x,y,L1,L2)
theta1 = atan(-x/y);
if theta1 ~= 0
    d = x / (2*sin(theta1));
    theta2 = acos(d/L1);
else
    d = -y/2;
    theta2 = acos(d/L1);
end
end

== matlab function t06_manual_control_sol/TURN LEFT GAIT/Plane Movement Right1/MATLAB Function2 ==
  data: x output; t input; Tdur input; y output; P0x input; P0z input; P1x input; P1z input; P2x input; P2z input; P3x input; P3z input
function [x, y] = bez_plane_TrajV2(t,Tdur,P0x,P0z,P1x,P1z,P2x,P2z,P3x,P3z)
t_swing = Tdur/4;
t_support = Tdur*3/4;

P0 = [P0x, P0z];
P1 = [P1x, P1z];
P2 = [P2x, P2z];
P3 = [P3x, P3z];
P_ini = (P0 + P3)/2;

if Tdur == 0
    x = -P_ini(1);
    y = P_ini(2);

elseif t<=t_support/2
    x = -1*(P_ini(1)+(P0(1)-P3(1))/t_support*(t));
    y = P_ini(2);

elseif t<=t_support/2+t_swing
    t_ef = (t-t_support/2);
    Sw = P0*((1-(t_ef/t_swing))^3) + 3*P1*(t_ef/t_swing)*((1-(t_ef/t_swing))^2)...
        + 3*P2*((t_ef/t_swing)^2)*(1-(t_ef/t_swing)) + P3*((t_ef/t_swing)^3);
    
    x = -1*Sw(1);
    y = Sw(2);
else
    t_ef = (t-t_support/2-t_swing);
    x = -1*(P3(1)+(P0(1)-P3(1))/t_support*t_ef);
    y = P0(2);
end

end

== matlab function t06_manual_control_sol/TURN RIGHT GAIT/Plane Movement Right1/MATLAB Function1 ==
  data: x input; theta1 output; y input; L1 input; L2 input; theta2 output
function [theta1, theta2] = angSide(x,y,L1,L2)
theta1 = atan(-x/y);
if theta1 ~= 0
    d = x / (2*sin(theta1));
    theta2 = acos(d/L1);
else
    d = -y/2;
    theta2 = acos(d/L1);
end
end

== matlab function t06_manual_control_sol/TURN LEFT GAIT/Plane Movement Left1/MATLAB Function ==
  data: x input; theta1Ad output; L1 input; L2 input; theta1 input
function theta1Ad = angAd(x, L1, L2, theta1)

l = cos(theta1)*(L1 + L2);

theta1Ad = asin(-x/l);

== matlab function t06_manual_control_sol/TURN LEFT GAIT/Plane Movement Left1/MATLAB Function1 ==
  data: x input; theta1 output; y input; L1 input; L2 input; theta2 output
function [theta1, theta2] = angSide(x,y,L1,L2)
theta1 = atan(-x/y);
if theta1 ~= 0
    d = x / (2*sin(theta1));
    theta2 = acos(d/L1);
else
    d = -y/2;
    theta2 = acos(d/L1);
end
end

== matlab function t06_manual_control_sol/TURN LEFT GAIT/Plane Movement Left1/MATLAB Function3 ==
  data: x output; t input; Tdur input; y output; P0x input; P0z input; P1x input; P1z input; P2x input; P2z input; P3x input; P3z input
function [x, y] = bez_plane_TrajV2(t,Tdur,P0x,P0z,P1x,P1z,P2x,P2z,P3x,P3z)
t_swing = Tdur/4;
t_support = Tdur*3/4;

P0 = [P0x, P0z];
P1 = [P1x, P1z];
P2 = [P2x, P2z];
P3 = [P3x, P3z];
P_ini = (P0 + P3)/2;

if Tdur == 0
    x = -P_ini(1);
    y = P_ini(2);

elseif t<=t_support/2
    x = -1*(P_ini(1)+(P3(1)-P0(1))/t_support*(t));
    y = P_ini(2);

elseif t<=t_support/2+t_swing
    t_ef = (t-t_support/2);
    Sw = P3*((1-(t_ef/t_swing))^3) + 3*P2*(t_ef/t_swing)*((1-(t_ef/t_swing))^2)...
        + 3*P1*((t_ef/t_swing)^2)*(1-(t_ef/t_swing)) + P0*((t_ef/t_swing)^3);
    
    x = -1*Sw(1);
    y = Sw(2);
else
    t_ef = (t-t_support/2-t_swing);
    x = -1*(P0(1)+(P3(1)-P0(1))/t_support*t_ef);
    y = P0(2);
end
end

== matlab function t06_manual_control_sol/Walk Back Gait - Bezier Curves/Plane Movement FL/MATLAB ==
  data: x input; theta1 output; y input; L1 input; L2 input; theta2 output
function [theta1, theta2] = ang(x,y,L1,L2)
x;
y;
(x.^2+y.^2-L1.^2-L2.^2) / (2*L1*L2);
theta2 = acos((x.^2+y.^2-L1.^2-L2.^2) / (2*L1*L2));
beta = asin((L2*sin(theta2))./((x.^2+y.^2).^0.5));
theta1 = asin(x./((x.^2+y.^2).^0.5)) + beta;
end

== matlab function t06_manual_control_sol/Walk Back Gait - Bezier Curves/Plane Movement FL/MATLAB Function ==
  data: y input; theta3 output; L1 input; L2 input; theta1 input; theta2 input
function theta3 = latAng(y, L1, L2, theta1, theta2)

l = cos(theta1)*(L1 + L2*cos(theta2));

theta3 = asin(y/l);

== matlab function t06_manual_control_sol/WALK FORWARD GAIT/Plane Movement Forward1/Longitudinal angles ==
  data: x input; theta1 output; y input; L1 input; L2 input; theta2 output
function [theta1, theta2] = ang(x,y,L1,L2)
x;
y;
(x.^2+y.^2-L1.^2-L2.^2) / (2*L1*L2);
theta2 = acos((x.^2+y.^2-L1.^2-L2.^2) / (2*L1*L2));
beta = asin((L2*sin(theta2))./((x.^2+y.^2).^0.5));
theta1 = asin(x./((x.^2+y.^2).^0.5)) + beta;
end

== matlab function t06_manual_control_sol/WALK FORWARD GAIT/Plane Movement Forward1/MATLAB Function2 ==
  data: x output; t input; Tdur input; y output; P0x input; P0z input; P1x input; P1z input; P2x input; P2z input; P3x input; P3z input
function [x, y] = bez_plane_TrajV2(t,Tdur,P0x,P0z,P1x,P1z,P2x,P2z,P3x,P3z)
t_swing = Tdur/4;
t_support = Tdur*3/4;

P0 = [P0x, P0z];
P1 = [P1x, P1z];
P2 = [P2x, P2z];
P3 = [P3x, P3z];
P_ini = (P0 + P3)/2;

if Tdur == 0
    x = -P_ini(1);
    y = P_ini(2);

elseif t<=t_support/2
    x = -1*(P_ini(1)+(P0(1)-P3(1))/t_support*(t));
    y = P_ini(2);

elseif t<=t_support/2+t_swing
    t_ef = (t-t_support/2);
    Sw = P0*((1-(t_ef/t_swing))^3) + 3*P1*(t_ef/t_swing)*((1-(t_ef/t_swing))^2)...
        + 3*P2*((t_ef/t_swing)^2)*(1-(t_ef/t_swing)) + P3*((t_ef/t_swing)^3);
    
    x = -1*Sw(1);
    y = Sw(2);
else
    t_ef = (t-t_support/2-t_swing);
    x = -1*(P3(1)+(P0(1)-P3(1))/t_support*t_ef);
    y = P0(2);
end

end

== matlab function t06_manual_control_sol/WALK FORWARD GAIT/Plane Movement Forward2/Lateral angles ==
  data: y input; theta3 output; L1 input; L2 input; theta1 input; theta2 input
function theta3 = latAng(y, L1, L2, theta1, theta2)

l = cos(theta1)*(L1 + L2*cos(theta2));

theta3 = asin(y/l);

== matlab function t06_manual_control_sol/WALK FORWARD GAIT/Plane Movement Forward2/Longitudinal angles ==
  data: x input; theta1 output; y input; L1 input; L2 input; theta2 output
function [theta1, theta2] = ang(x,y,L1,L2)
x;
y;
(x.^2+y.^2-L1.^2-L2.^2) / (2*L1*L2);
theta2 = acos((x.^2+y.^2-L1.^2-L2.^2) / (2*L1*L2));
beta = asin((L2*sin(theta2))./((x.^2+y.^2).^0.5));
theta1 = asin(x./((x.^2+y.^2).^0.5)) + beta;
end

== matlab function t06_manual_control_sol/TURN RIGHT GAIT/Plane Movement Right1/MATLAB Function2 ==
  data: x output; t input; Tdur input; y output; P0x input; P0z input; P1x input; P1z input; P2x input; P2z input; P3x input; P3z input
function [x, y] = bez_plane_TrajV2(t,Tdur,P0x,P0z,P1x,P1z,P2x,P2z,P3x,P3z)
t_swing = Tdur/4;
t_support = Tdur*3/4;

P0 = [P0x, P0z];
P1 = [P1x, P1z];
P2 = [P2x, P2z];
P3 = [P3x, P3z];
P_ini = (P0 + P3)/2;

if Tdur == 0
    x = -P_ini(1);
    y = P_ini(2);

elseif t<=t_support/2
    x = -1*(P_ini(1)+(P0(1)-P3(1))/t_support*(t));
    y = P_ini(2);

elseif t<=t_support/2+t_swing
    t_ef = (t-t_support/2);
    Sw = P0*((1-(t_ef/t_swing))^3) + 3*P1*(t_ef/t_swing)*((1-(t_ef/t_swing))^2)...
        + 3*P2*((t_ef/t_swing)^2)*(1-(t_ef/t_swing)) + P3*((t_ef/t_swing)^3);
    
    x = -1*Sw(1);
    y = Sw(2);
else
    t_ef = (t-t_support/2-t_swing);
    x = -1*(P3(1)+(P0(1)-P3(1))/t_support*t_ef);
    y = P0(2);
end

end

== matlab function t06_manual_control_sol/WALK FORWARD GAIT/Plane Movement Forward2/MATLAB Function2 ==
  data: x output; t input; Tdur input; y output; P0x input; P0z input; P1x input; P1z input; P2x input; P2z input; P3x input; P3z input
function [x, y] = bez_plane_TrajV2(t,Tdur,P0x,P0z,P1x,P1z,P2x,P2z,P3x,P3z)
t_swing = Tdur/4;
t_support = Tdur*3/4;

P0 = [P0x, P0z];
P1 = [P1x, P1z];
P2 = [P2x, P2z];
P3 = [P3x, P3z];
P_ini = (P0 + P3)/2;

if Tdur == 0
    x = -P_ini(1);
    y = P_ini(2);

elseif t<=t_support/2
    x = -1*(P_ini(1)+(P0(1)-P3(1))/t_support*(t));
    y = P_ini(2);

elseif t<=t_support/2+t_swing
    t_ef = (t-t_support/2);
    Sw = P0*((1-(t_ef/t_swing))^3) + 3*P1*(t_ef/t_swing)*((1-(t_ef/t_swing))^2)...
        + 3*P2*((t_ef/t_swing)^2)*(1-(t_ef/t_swing)) + P3*((t_ef/t_swing)^3);
    
    x = -1*Sw(1);
    y = Sw(2);
else
    t_ef = (t-t_support/2-t_swing);
    x = -1*(P3(1)+(P0(1)-P3(1))/t_support*t_ef);
    y = P0(2);
end

end

== matlab function t06_manual_control_sol/WALK FORWARD GAIT/Plane Movement Forward3/Lateral angles ==
  data: y input; theta3 output; L1 input; L2 input; theta1 input; theta2 input
function theta3 = latAng(y, L1, L2, theta1, theta2)

l = cos(theta1)*(L1 + L2*cos(theta2));

theta3 = asin(y/l);

== matlab function t06_manual_control_sol/WALK FORWARD GAIT/Plane Movement Forward3/Longitudinal angles ==
  data: x input; theta1 output; y input; L1 input; L2 input; theta2 output
function [theta1, theta2] = ang(x,y,L1,L2)
x;
y;
(x.^2+y.^2-L1.^2-L2.^2) / (2*L1*L2);
theta2 = acos((x.^2+y.^2-L1.^2-L2.^2) / (2*L1*L2));
beta = asin((L2*sin(theta2))./((x.^2+y.^2).^0.5));
theta1 = asin(x./((x.^2+y.^2).^0.5)) + beta;
end

== matlab function t06_manual_control_sol/WALK FORWARD GAIT/Plane Movement Forward3/MATLAB Function2 ==
  data: x output; t input; Tdur input; y output; P0x input; P0z input; P1x input; P1z input; P2x input; P2z input; P3x input; P3z input
function [x, y] = bez_plane_TrajV2(t,Tdur,P0x,P0z,P1x,P1z,P2x,P2z,P3x,P3z)
t_swing = Tdur/4;
t_support = Tdur*3/4;

P0 = [P0x, P0z];
P1 = [P1x, P1z];
P2 = [P2x, P2z];
P3 = [P3x, P3z];
P_ini = (P0 + P3)/2;

if Tdur == 0
    x = -P_ini(1);
    y = P_ini(2);

elseif t<=t_support/2
    x = -1*(P_ini(1)+(P0(1)-P3(1))/t_support*(t));
    y = P_ini(2);

elseif t<=t_support/2+t_swing
    t_ef = (t-t_support/2);
    Sw = P0*((1-(t_ef/t_swing))^3) + 3*P1*(t_ef/t_swing)*((1-(t_ef/t_swing))^2)...
        + 3*P2*((t_ef/t_swing)^2)*(1-(t_ef/t_swing)) + P3*((t_ef/t_swing)^3);
    
    x = -1*Sw(1);
    y = Sw(2);
else
    t_ef = (t-t_support/2-t_swing);
    x = -1*(P3(1)+(P0(1)-P3(1))/t_support*t_ef);
    y = P0(2);
end

end

== matlab function t06_manual_control_sol/TURN LEFT GAIT/Plane Movement Left/MATLAB Function ==
  data: x input; theta1Ad output; L1 input; L2 input; theta1 input
function theta1Ad = angAd(x, L1, L2, theta1)

l = cos(theta1)*(L1 + L2);

theta1Ad = asin(-x/l);

== matlab function t06_manual_control_sol/TURN LEFT GAIT/Plane Movement Left/MATLAB Function1 ==
  data: x input; theta1 output; y input; L1 input; L2 input; theta2 output
function [theta1, theta2] = angSide(x,y,L1,L2)
theta1 = atan(-x/y);
if theta1 ~= 0
    d = x / (2*sin(theta1));
    theta2 = acos(d/L1);
else
    d = -y/2;
    theta2 = acos(d/L1);
end
end

== matlab function t06_manual_control_sol/TURN LEFT GAIT/Plane Movement Left/MATLAB Function3 ==
  data: x output; t input; Tdur input; y output; P0x input; P0z input; P1x input; P1z input; P2x input; P2z input; P3x input; P3z input
function [x, y] = bez_plane_TrajV2(t,Tdur,P0x,P0z,P1x,P1z,P2x,P2z,P3x,P3z)
t_swing = Tdur/4;
t_support = Tdur*3/4;

P0 = [P0x, P0z];
P1 = [P1x, P1z];
P2 = [P2x, P2z];
P3 = [P3x, P3z];
P_ini = (P0 + P3)/2;

if Tdur == 0
    x = -P_ini(1);
    y = P_ini(2);

elseif t<=t_support/2
    x = -1*(P_ini(1)+(P3(1)-P0(1))/t_support*(t));
    y = P_ini(2);

elseif t<=t_support/2+t_swing
    t_ef = (t-t_support/2);
    Sw = P3*((1-(t_ef/t_swing))^3) + 3*P2*(t_ef/t_swing)*((1-(t_ef/t_swing))^2)...
        + 3*P1*((t_ef/t_swing)^2)*(1-(t_ef/t_swing)) + P0*((t_ef/t_swing)^3);
    
    x = -1*Sw(1);
    y = Sw(2);
else
    t_ef = (t-t_support/2-t_swing);
    x = -1*(P0(1)+(P3(1)-P0(1))/t_support*t_ef);
    y = P0(2);
end
end

== matlab function t06_manual_control_sol/TURN LEFT GAIT/Plane Movement Right/MATLAB Function ==
  data: x input; theta1Ad output; L1 input; L2 input; theta1 input
function theta1Ad = angAd(x, L1, L2, theta1)

l = cos(theta1)*(L1 + L2);

theta1Ad = asin(-x/l);

== matlab function t06_manual_control_sol/TURN LEFT GAIT/Plane Movement Right/MATLAB Function1 ==
  data: x input; theta1 output; y input; L1 input; L2 input; theta2 output
function [theta1, theta2] = angSide(x,y,L1,L2)
theta1 = atan(-x/y);
if theta1 ~= 0
    d = x / (2*sin(theta1));
    theta2 = acos(d/L1);
else
    d = -y/2;
    theta2 = acos(d/L1);
end
end

== matlab function t06_manual_control_sol/TURN LEFT GAIT/Plane Movement Right/MATLAB Function2 ==
  data: x output; t input; Tdur input; y output; P0x input; P0z input; P1x input; P1z input; P2x input; P2z input; P3x input; P3z input
function [x, y] = bez_plane_TrajV2(t,Tdur,P0x,P0z,P1x,P1z,P2x,P2z,P3x,P3z)
t_swing = Tdur/4;
t_support = Tdur*3/4;

P0 = [P0x, P0z];
P1 = [P1x, P1z];
P2 = [P2x, P2z];
P3 = [P3x, P3z];
P_ini = (P0 + P3)/2;

if Tdur == 0
    x = -P_ini(1);
    y = P_ini(2);

elseif t<=t_support/2
    x = -1*(P_ini(1)+(P0(1)-P3(1))/t_support*(t));
    y = P_ini(2);

elseif t<=t_support/2+t_swing
    t_ef = (t-t_support/2);
    Sw = P0*((1-(t_ef/t_swing))^3) + 3*P1*(t_ef/t_swing)*((1-(t_ef/t_swing))^2)...
        + 3*P2*((t_ef/t_swing)^2)*(1-(t_ef/t_swing)) + P3*((t_ef/t_swing)^3);
    
    x = -1*Sw(1);
    y = Sw(2);
else
    t_ef = (t-t_support/2-t_swing);
    x = -1*(P3(1)+(P0(1)-P3(1))/t_support*t_ef);
    y = P0(2);
end

end

== matlab function t06_manual_control_sol/TURN RIGHT GAIT/Plane Movement Left/MATLAB Function ==
  data: x input; theta1Ad output; L1 input; L2 input; theta1 input
function theta1Ad = angAd(x, L1, L2, theta1)

l = cos(theta1)*(L1 + L2);

theta1Ad = asin(-x/l);

== matlab function t06_manual_control_sol/TURN RIGHT GAIT/Plane Movement Left/MATLAB Function1 ==
  data: x input; theta1 output; y input; L1 input; L2 input; theta2 output
function [theta1, theta2] = angSide(x,y,L1,L2)
theta1 = atan(-x/y);
if theta1 ~= 0
    d = x / (2*sin(theta1));
    theta2 = acos(d/L1);
else
    d = -y/2;
    theta2 = acos(d/L1);
end
end

== matlab function t06_manual_control_sol/TURN RIGHT GAIT/Plane Movement Left/MATLAB Function3 ==
  data: x output; t input; Tdur input; y output; P0x input; P0z input; P1x input; P1z input; P2x input; P2z input; P3x input; P3z input
function [x, y] = bez_plane_TrajV2(t,Tdur,P0x,P0z,P1x,P1z,P2x,P2z,P3x,P3z)
t_swing = Tdur/4;
t_support = Tdur*3/4;

P0 = [P0x, P0z];
P1 = [P1x, P1z];
P2 = [P2x, P2z];
P3 = [P3x, P3z];
P_ini = (P0 + P3)/2;

if Tdur == 0
    x = -P_ini(1);
    y = P_ini(2);

elseif t<=t_support/2
    x = -1*(P_ini(1)+(P3(1)-P0(1))/t_support*(t));
    y = P_ini(2);

elseif t<=t_support/2+t_swing
    t_ef = (t-t_support/2);
    Sw = P3*((1-(t_ef/t_swing))^3) + 3*P2*(t_ef/t_swing)*((1-(t_ef/t_swing))^2)...
        + 3*P1*((t_ef/t_swing)^2)*(1-(t_ef/t_swing)) + P0*((t_ef/t_swing)^3);
    
    x = -1*Sw(1);
    y = Sw(2);
else
    t_ef = (t-t_support/2-t_swing);
    x = -1*(P0(1)+(P3(1)-P0(1))/t_support*t_ef);
    y = P0(2);
end
end

== matlab function t06_manual_control_sol/WALK FORWARD GAIT/Plane Movement Forward/Lateral angles ==
  data: y input; theta3 output; L1 input; L2 input; theta1 input; theta2 input
function theta3 = latAng(y, L1, L2, theta1, theta2)

l = cos(theta1)*(L1 + L2*cos(theta2));

theta3 = asin(y/l);

== matlab function t06_manual_control_sol/TURN RIGHT GAIT/Plane Movement Right/MATLAB Function ==
  data: x input; theta1Ad output; L1 input; L2 input; theta1 input
function theta1Ad = angAd(x, L1, L2, theta1)

l = cos(theta1)*(L1 + L2);

theta1Ad = asin(-x/l);

== matlab function t06_manual_control_sol/TURN RIGHT GAIT/Plane Movement Right/MATLAB Function1 ==
  data: x input; theta1 output; y input; L1 input; L2 input; theta2 output
function [theta1, theta2] = angSide(x,y,L1,L2)
theta1 = atan(-x/y);
if theta1 ~= 0
    d = x / (2*sin(theta1));
    theta2 = acos(d/L1);
else
    d = -y/2;
    theta2 = acos(d/L1);
end
end

== matlab function t06_manual_control_sol/TURN RIGHT GAIT/Plane Movement Right/MATLAB Function2 ==
  data: x output; t input; Tdur input; y output; P0x input; P0z input; P1x input; P1z input; P2x input; P2z input; P3x input; P3z input
function [x, y] = bez_plane_TrajV2(t,Tdur,P0x,P0z,P1x,P1z,P2x,P2z,P3x,P3z)
t_swing = Tdur/4;
t_support = Tdur*3/4;

P0 = [P0x, P0z];
P1 = [P1x, P1z];
P2 = [P2x, P2z];
P3 = [P3x, P3z];
P_ini = (P0 + P3)/2;

if Tdur == 0
    x = -P_ini(1);
    y = P_ini(2);

elseif t<=t_support/2
    x = -1*(P_ini(1)+(P0(1)-P3(1))/t_support*(t));
    y = P_ini(2);

elseif t<=t_support/2+t_swing
    t_ef = (t-t_support/2);
    Sw = P0*((1-(t_ef/t_swing))^3) + 3*P1*(t_ef/t_swing)*((1-(t_ef/t_swing))^2)...
        + 3*P2*((t_ef/t_swing)^2)*(1-(t_ef/t_swing)) + P3*((t_ef/t_swing)^3);
    
    x = -1*Sw(1);
    y = Sw(2);
else
    t_ef = (t-t_support/2-t_swing);
    x = -1*(P3(1)+(P0(1)-P3(1))/t_support*t_ef);
    y = P0(2);
end

end

== matlab function t06_manual_control_sol/Walk Back Gait - Bezier Curves/Plane Movement FL/MATLAB Function2 ==
  data: x output; t input; Tdur input; y output; P0x input; P0z input; P1x input; P1z input; P2x input; P2z input; P3x input; P3z input
function [x, y] = bez_plane_TrajV2(t,Tdur,P0x,P0z,P1x,P1z,P2x,P2z,P3x,P3z)
t_swing = Tdur/4;
t_support = Tdur*3/4;

P0 = [P0x, P0z];
P1 = [P1x, P1z];
P2 = [P2x, P2z];
P3 = [P3x, P3z];
P_ini = (P0 + P3)/2;

if Tdur == 0
    x = -P_ini(1);
    y = P_ini(2);

elseif t<=t_support/2
    x = -1*(P_ini(1)+(P3(1)-P0(1))/t_support*(t));
    y = P_ini(2);

elseif t<=t_support/2+t_swing
    t_ef = (t-t_support/2);
    Sw = P3*((1-(t_ef/t_swing))^3) + 3*P2*(t_ef/t_swing)*((1-(t_ef/t_swing))^2)...
        + 3*P1*((t_ef/t_swing)^2)*(1-(t_ef/t_swing)) + P0*((t_ef/t_swing)^3);
    
    x = -1*Sw(1);
    y = Sw(2);
else
    t_ef = (t-t_support/2-t_swing);
    x = -1*(P0(1)+(P3(1)-P0(1))/t_support*t_ef);
    y = P0(2);
end
end
